simulink model "test_sim2"  (R2022b)
settings: Solver=ode4  StartTime=0.0  StopTime=30.0  FixedStep=0.001  RelTol=1e-3
values from neighbouring files (symbols this model uses):
  a = 10    [paraset.m]
  b = 4    [paraset.m]
settings Model: Creator=user  LastModifiedBy=user
settings DataIOCC: ReturnWorkspaceOutputs=off

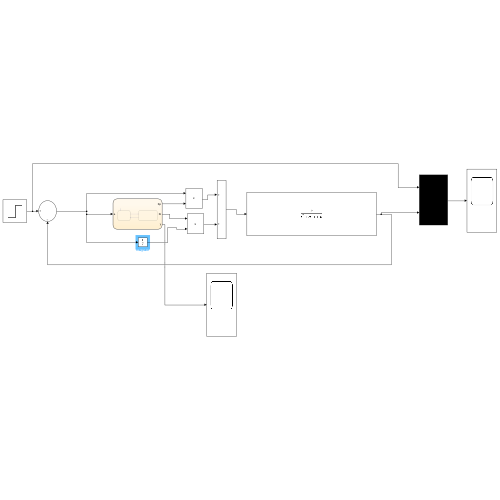
[thumbnail: Simulink's stored preview of the top-level diagram]
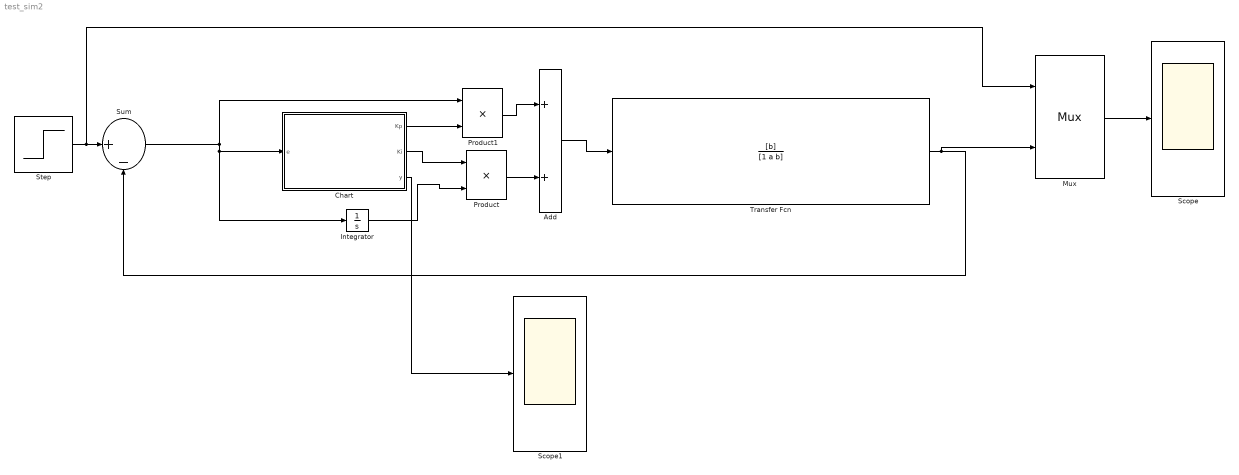
== system test_sim2 ==
  Add : Sum
  Chart : Stateflow chart  TreatAsAtomicUnit=on
  Integrator : Integrator
  Mux : Mux  Inputs=2
  Product : Product
  Product1 : Product
  Scope : Scope
  Scope1 : Scope
  Step : Step  SampleTime=0
  Sum : Sum  Inputs=|+-
  Transfer Fcn : TransferFcn  Numerator=[b]  Denominator=[1 a b]
  wires:
  Transfer Fcn/1 -> Mux/2, Sum/2
  Step/1 -> Mux/1, Sum/1
  Mux/1 -> Scope/1
  Sum/1 -> Integrator/1, Chart/1(e), Product1/1
  Integrator/1 -> Product/2
  Chart/2(Ki) -> Product/1
  Chart/1(Kp) -> Product1/2
  Product1/1 -> Add/1
  Product/1 -> Add/2
  Add/1 -> Transfer Fcn/1
  Chart/3(y) -> Scope1/1

== stateflow chart test_sim2/Chart ==
  state PID1
    Kp = 0.5
    Ki = 0.9
    y=1
  state PID2
    Kp = 1
    Ki = 2
    y=2
  (default) -> PID1
  PID1 -> PID2 : [abs(e)>0.1]
  PID2 -> PID1 : [abs(e)<=0.1]
  data: e input; Kp output; Ki output; y output
